simulink model "augmented_sgp4_exp"  (R2018a)
settings: Solver=VariableStepAuto  StartTime=0.0  StopTime=sim_stop  RelTol=1e-3
settings Model: Creator=Yashren  LastModifiedBy=Yashren

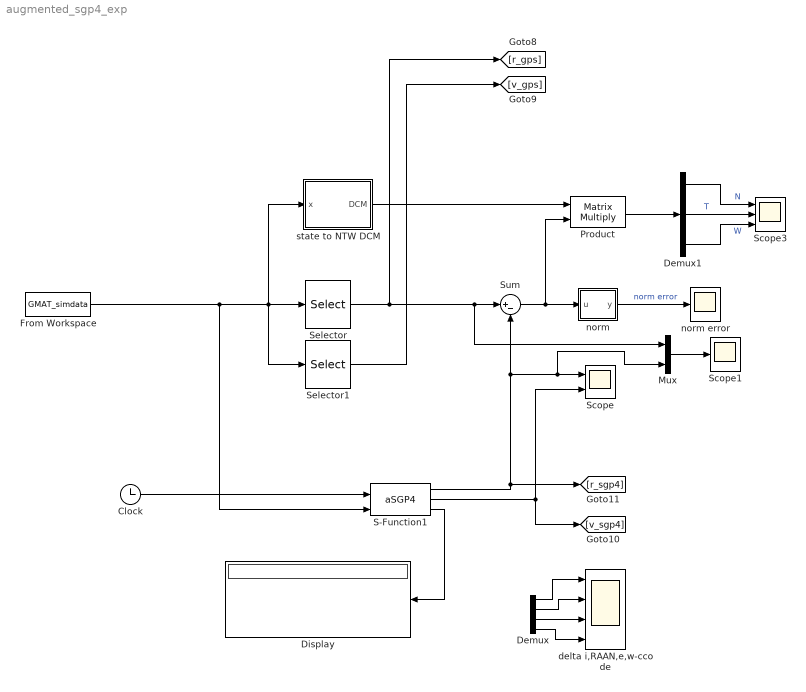
== system augmented_sgp4_exp ==
  Clock : Clock
  Demux : Demux
  Demux1 : Demux  Outputs=3
  Display : Display
      settings: Format=long_e
  From Workspace : FromWorkspace  VariableName=GMAT_simdata
  Mux : Mux  Inputs=2
  Product : Product  Multiplication=Matrix(*)
  S-Function1 : S-Function  FunctionName=aSGP4  Parameters=orbit_start_UTC  SFunctionDeploymentMode=off  EnableBusSupport=off
  Scope : Scope  NumInputPorts=2
  Scope1 : Scope
  Scope3 : Scope  NumInputPorts=3
  Selector : Selector  InputPortWidth=6  IndexOptions=Index vector (dialog)  Indices=[1 2 3]  OutputSizes=1
  Selector1 : Selector  InputPortWidth=6  IndexOptions=Index vector (dialog)  Indices=[4 5 6]  OutputSizes=1
  Sum : Sum  Inputs=|+-
  delta i,RAAN,e,w-ccode : Scope  NumInputPorts=4
  norm : Subsystem
  norm error : Scope
  state to NTW DCM : MATLAB Function  TreatAsAtomicUnit=on
  wires:
  Clock/1 -> S-Function1/1
  S-Function1/2 -> [v_sgp4], Scope/2
  Mux/1 -> Scope1/1
  Selector/1 -> [r_gps], Mux/1, Sum/1
  state to NTW DCM/1(DCM) -> Product/1
  Sum/1 -> Product/2, norm/1(u)
  norm/1(y) -> norm error/1  "norm error"
  Selector1/1 -> [v_gps]
  S-Function1/1 -> [r_sgp4], Sum/2, Mux/2, Scope/1
  Demux/3 -> delta i,RAAN,e,w-ccode/3
  Demux/2 -> delta i,RAAN,e,w-ccode/2
  Demux/4 -> delta i,RAAN,e,w-ccode/4
  Demux/1 -> delta i,RAAN,e,w-ccode/1
  Product/1 -> Demux1/1
  Demux1/1 -> Scope3/1  "N"
  Demux1/2 -> Scope3/2  "T"
  Demux1/3 -> Scope3/3  "W"
  From Workspace/1 -> S-Function1/2, Selector1/1, Selector/1, state to NTW DCM/1(x)
  S-Function1/3 -> Display/1

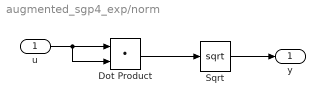
== system augmented_sgp4_exp/norm ==
  u : Inport
  Dot Product : DotProduct  InputSameDT=on  OutDataTypeStr=Inherit: Inherit via internal rule
  Sqrt : Sqrt  SaturateOnIntegerOverflow=on
  y : Outport
  wires:
  u/1 -> Dot Product/2, Dot Product/1
  Dot Product/1 -> Sqrt/1
  Sqrt/1 -> y/1

== matlab function augmented_sgp4_exp/state to NTW DCM ==
  data: x input; DCM output
function DCM = fcn(x)

% function takes in satellite state r,v
% generates DCM to convert ECI to NTW
r = x(1:3);
v = x(4:6);
T = v/norm(v);
W = cross(r,v);
W = W/norm(W);
N = cross(T,W);

DCM = [N,T,W]';
